simulink model "Pnormtrail1"  (Simulink 8.1)
settings: Solver=ode45  StartTime=0.0  StopTime=1000  RelTol=1e-3
libraries: commchan3 x1, commdigbbndpm3 x1, commrandsrc2 x1, simulink x1
settings Model: Creator=Gaurav  LastModifiedBy=Gaurav
settings DataIOCC: SignalLoggingSaveFormat=Dataset
settings OptimizationCC: ExpressionDepthLimit=128
settings DebuggingCC: FcnCallInpInsideContextMsg=EnableAllAsError
settings GRTTargetCC: CombineOutputUpdateFcns=on  GRTInterface=off

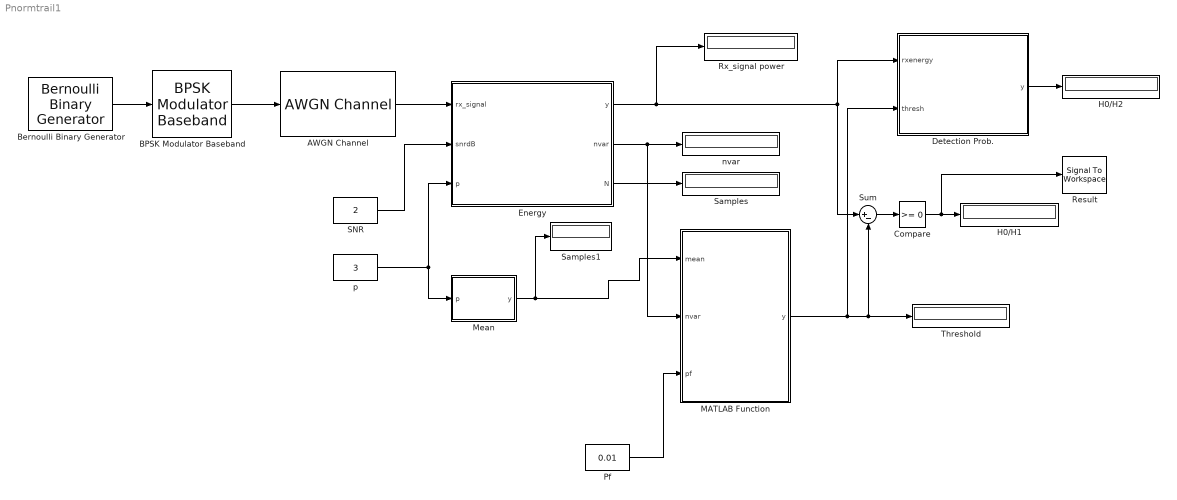
== system Pnormtrail1 ==
  AWGN Channel : commchan3/AWGN Channel  InputProcessing=Columns as channels (frame based)  seed=67  noiseMode="Signal to noise ratio  (SNR)"  EbNodB=10  EsNodB=10  SNRdB=-8  bitsPerSym=1  Ps=1  Tsym=1  variance=1
  BPSK Modulator Baseband : commdigbbndpm3/BPSK Modulator Baseband  Ph=0  outDtype=double  outWordLen=16  outUDDataType=sfix(16)  outFracLenMode=Best precision  outFracLen=15
  Bernoulli Binary Generator : commrandsrc2/Bernoulli Binary Generator  P=0.5  seed=90  Ts=0.01  frameBased=on  sampPerFrame=100  orient=off  outDataType=double
  Compare : simulink/Logic and Bit Operations/Compare To Zero  relop=>=  OutDataTypeStr=boolean
  Detection Prob. : MATLAB Function  TreatAsAtomicUnit=on
  Energy : MATLAB Function  TreatAsAtomicUnit=on
  H0/H1 : Display
  H0/H2 : Display
  MATLAB Function : MATLAB Function  TreatAsAtomicUnit=on
  Mean : MATLAB Function  TreatAsAtomicUnit=on
  Pf : Constant  Value=0.01
  Result : SignalToWorkspace  VariableName=Stat
      settings: CopyFcn=dspblkcopystw(gcbh);
  Rx_signal power : Display
  SNR : Constant  Value=2
  Samples : Display
  Samples1 : Display
  Sum : Sum  Inputs=|+-
  Threshold : Display
  nvar : Display
  p : Constant  Value=3
  wires:
  Bernoulli Binary Generator/1 -> BPSK Modulator Baseband/1
  BPSK Modulator Baseband/1 -> AWGN Channel/1
  AWGN Channel/1 -> Energy/1(rx_signal)
  SNR/1 -> Energy/2(snrdB)
  Energy/1(y) -> Rx_signal power/1, Detection Prob./1(rxenergy), Sum/1
  Energy/2(nvar) -> MATLAB Function/2(nvar), nvar/1
  Energy/3(N) -> Samples/1
  MATLAB Function/1(y) -> Detection Prob./2(thresh), Threshold/1, Sum/2
  Sum/1 -> Compare/1
  Compare/1 -> Result/1, H0/H1/1
  Detection Prob./1(y) -> H0/H2/1
  p/1 -> Mean/1(p), Energy/3(p)
  Mean/1(y) -> MATLAB Function/1(mean), Samples1/1
  Pf/1 -> MATLAB Function/3(pf)

== matlab function MATLAB Function ==
  data: mean input double; y output double; nvar input double; pf input double
function y = Threshold(mean,nvar,pf)
    coder.extrinsic('qfuncinv');
    t=double(zeros(1,1));
    t=qfuncinv(pf);
    thresh=double(zeros(1,1));
    thresh = nvar.*t + mean;
y=thresh;

== matlab function Energy ==
  data: rx_signal input double; y output double; snrdB input double; nvar output double; N output double; p input double
function [y,nvar,N] = Energy(rx_signal,snrdB,p)
    [n,m]=size(rx_signal);
    snr = 10^(snrdB/20);
    nvar = 1/snr;                               % noise variance
    %energy=double(zeros(1,1));
    energy = sum((abs(rx_signal).^p));
    power= (energy)./1000;
    y = power;
    N=n;

== matlab function Detection Prob. ==
  data: rxenergy input double; y output double; thresh input double
function y = Detectionprob(rxenergy,thresh)
       t=double(zeros(1,1));
       if(rxenergy>=thresh)
           t=t+1;
       end
%     [p q]=size(R);
%     detect=double(zeros(1,1));
%     for i=1:p
%         p
%         if(R(p,1)==1)
%             detect=detect+1;
%             detect
%         end
%     end
y = t;

== matlab function Mean ==
  data: p input double; y output double
function y = Mean(p)
coder.extrinsic('gamma');
b=double(zeros(1,1));
a=2.^(p/2);
b=gamma((p+1)/2);
mu=(a/1.775).*b;
y = mu;
